simulink model "DYNctl_ver4_etud_obfusc"  (R2018b)
settings: Solver=ode45  StartTime=0.0  StopTime=tfin  FixedStep=0.001  RelTol=1e-09  EnableMultiTasking=on
values from neighbouring files (symbols this model uses):
  g = 9.81    [bancEssaiConstantes.m]
  JS = 2*mS*rS^2/5    (= 4.8672e-08)    [bancEssaiConstantes.m]
  Jxy = Jx    (= 0.001169)    [bancEssaiConstantes.m]
  L = LL    (= 0.115)    [bancEssaiConstantes.m]
  mP = 425e-03    (= 0.425)    [bancEssaiConstantes.m]
  mS = 0.0080    (= 0.008)    [bancEssaiConstantes.m]
  R = RR    (= 3.6)    [bancEssaiConstantes.m]
  rABC = 95.20e-03    (= 0.0952)    [bancEssaiConstantes.m]
  rS = 0.0039    [bancEssaiConstantes.m]
  XA = +rABC    (= 0.0952)    [bancEssaiConstantes.m]
  XB = -rABC*sind(30)    [bancEssaiConstantes.m]
  XC = -rABC*sind(30)    [bancEssaiConstantes.m]
  YA = 0.0    (= 0)    [bancEssaiConstantes.m]
  YB = +rABC*cosd(30)    [bancEssaiConstantes.m]
  YC = -rABC*cosd(30)    [bancEssaiConstantes.m]
undefined symbols (not defined in the file or in its folder): ae0, ae1, ae2, ae3, as0, as1, as2, as3, be1
settings Model: Creator=delafontaine  LastModifiedBy=Vincent
settings SolverCC: AlgebraicLoopSolver=LineSearch
settings DataIOCC: LimitDataPoints=on  SaveFormat=Array  SignalLoggingSaveFormat=ModelDataLogs
settings OptimizationCC: LifeSpan=inf
settings DebuggingCC: UnderspecifiedInitializationDetection=Classic  MergeDetectMultiDrivingBlocksExec=none  MultiTaskDSMMsg=warning  MultiTaskCondExecSysMsg=none  SFUnexpectedBacktrackingDiag=warning  SFNoUnconditionalDefaultTransitionDiag=warning  SFExecutionAtInitializationDiag=none
settings HardwareCC: ProdBitPerPointer=32  ProdBitPerSizeT=32  ProdBitPerPtrDiffT=32  ProdLargestAtomicFloat=None  ProdIntDivRoundTo=Undefined  ProdEndianess=Unspecified  ProdWordSize=32  ProdHWDeviceType=32-bit Generic
settings ModelReferenceCC: PropagateSignalLabelsOutOfModel=off
settings SFSimCC: SimUseLocalCustomCode=off
settings RTWCC: RTWUseLocalCustomCode=off
settings CodeAppCC: StateflowObjectComments=on
settings GRTTargetCC: TargetLangStandard=C89/C90 (ANSI)  GeneratePreprocessorConditionals=Disable all
settings ConfigComp: CovMetricSettings=dw  CovHtmlReporting=on  CovSaveCumulativeToWorkspaceVar=on  CovSaveSingleToWorkspaceVar=on  CovExternalEMLEnable=off  CovSFcnEnable=off

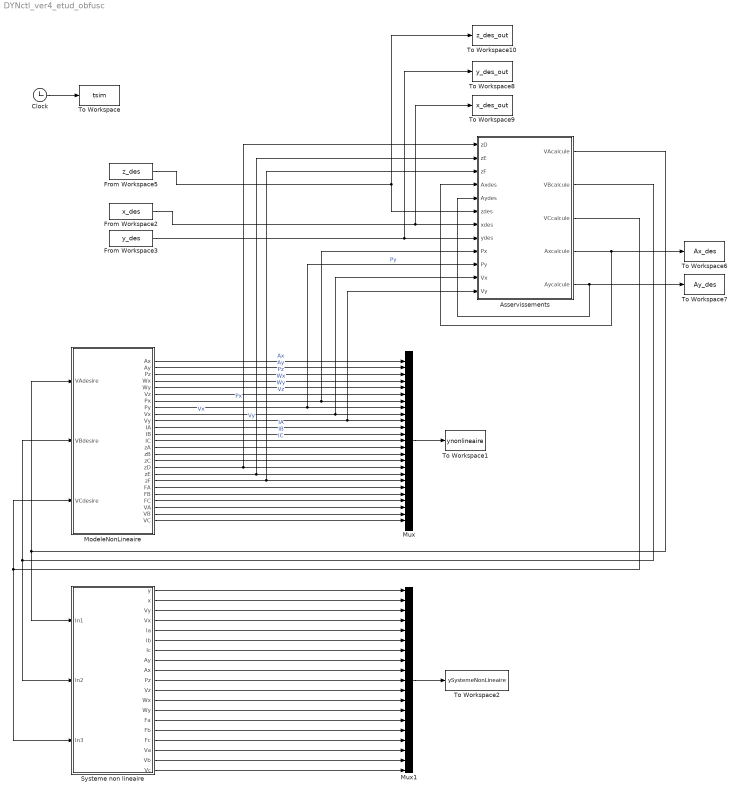
== system DYNctl_ver4_etud_obfusc ==
  Asservissements : Subsystem
      mask help: Simulink:masks:GenSFuncDesc_MD
      mask Help: eval('feval(''rtwprivate'',''rtwhelpview'',''rtw_sfcn_block'')');
  Clock : Clock
  From Workspace2 : FromWorkspace  VariableName=x_des  SampleTime=0  Interpolate=off  OutputAfterFinalValue=Holding final value
  From Workspace3 : FromWorkspace  VariableName=y_des  SampleTime=0  Interpolate=off  OutputAfterFinalValue=Holding final value
  From Workspace5 : FromWorkspace  VariableName=z_des  SampleTime=0  Interpolate=off  OutputAfterFinalValue=Holding final value
  ModeleNonLineaire : Subsystem
      mask help: Simulink:masks:GenSFuncDesc_MD
      mask Help: eval('feval(''rtwprivate'',''rtwhelpview'',''rtw_sfcn_block'')');
  Mux : Mux  Inputs=25
  Mux1 : Mux  Inputs=19
  Systeme non lineaire : Subsystem
  To Workspace : ToWorkspace  VariableName=tsim  SampleTime=-1
  To Workspace1 : ToWorkspace  VariableName=ynonlineaire  SampleTime=-1
  To Workspace10 : ToWorkspace  VariableName=z_des_out  SampleTime=-1
  To Workspace2 : ToWorkspace  VariableName=ySystemeNonLineaire  SampleTime=-1
  To Workspace6 : ToWorkspace  VariableName=Ax_des  SampleTime=-1
  To Workspace7 : ToWorkspace  VariableName=Ay_des  SampleTime=-1
  To Workspace8 : ToWorkspace  VariableName=y_des_out  SampleTime=-1
  To Workspace9 : ToWorkspace  VariableName=x_des_out  SampleTime=-1
  wires:
  Mux/1 -> To Workspace1/1
  Clock/1 -> To Workspace/1
  From Workspace5/1 -> Asservissements/6(zdes), To Workspace10/1
  ModeleNonLineaire/1(Ax) -> Mux/1  "Ax"
  ModeleNonLineaire/2(Ay) -> Mux/2  "Ay"
  ModeleNonLineaire/3(Pz) -> Mux/3  "Pz"
  ModeleNonLineaire/4(Wx) -> Mux/4  "Wx"
  ModeleNonLineaire/5(Wy) -> Mux/5  "Wy"
  ModeleNonLineaire/6(Vz) -> Mux/6  "Vz"
  ModeleNonLineaire/7(Px) -> Asservissements/9(Px), Mux/7  "Px"
  ModeleNonLineaire/8(Py) -> Asservissements/10(Py), Mux/8  "Py"
  ModeleNonLineaire/9(Vx) -> Asservissements/11(Vx), Mux/9  "Vx"
  ModeleNonLineaire/10(Vy) -> Asservissements/12(Vy), Mux/10  "Vy"
  ModeleNonLineaire/11(IA) -> Mux/11  "IA"
  ModeleNonLineaire/12(IB) -> Mux/12  "IB"
  ModeleNonLineaire/13(IC) -> Mux/13  "IC"
  From Workspace3/1 -> Asservissements/8(ydes), To Workspace8/1
  From Workspace2/1 -> Asservissements/7(xdes), To Workspace9/1
  ModeleNonLineaire/20(FA) -> Mux/20
  ModeleNonLineaire/21(FB) -> Mux/21
  ModeleNonLineaire/22(FC) -> Mux/22
  ModeleNonLineaire/23(VA) -> Mux/23
  ModeleNonLineaire/24(VB) -> Mux/24
  ModeleNonLineaire/25(VC) -> Mux/25
  ModeleNonLineaire/17(zD) -> Asservissements/1(zD), Mux/17
  ModeleNonLineaire/18(zE) -> Asservissements/2(zE), Mux/18
  ModeleNonLineaire/19(zF) -> Asservissements/3(zF), Mux/19
  ModeleNonLineaire/14(zA) -> Mux/14
  ModeleNonLineaire/15(zB) -> Mux/15
  ModeleNonLineaire/16(zC) -> Mux/16
  Asservissements/4(Axcalcule) -> Asservissements/4(Axdes), To Workspace6/1
  Asservissements/5(Aycalcule) -> Asservissements/5(Aydes), To Workspace7/1
  Asservissements/1(VAcalcule) -> Systeme non lineaire/1(In1), ModeleNonLineaire/1(VAdesire)
  Asservissements/2(VBcalcule) -> Systeme non lineaire/2(In2), ModeleNonLineaire/2(VBdesire)
  Asservissements/3(VCcalcule) -> ModeleNonLineaire/3(VCdesire), Systeme non lineaire/3(In3)
  Systeme non lineaire/4(Vx) -> Mux1/4
  Systeme non lineaire/3(Vy) -> Mux1/3
  Systeme non lineaire/2(x) -> Mux1/2
  Systeme non lineaire/1(y) -> Mux1/1
  Systeme non lineaire/5(Ia) -> Mux1/5
  Systeme non lineaire/6(Ib) -> Mux1/6
  Systeme non lineaire/7(Ic) -> Mux1/7
  Systeme non lineaire/8(Ay) -> Mux1/8
  Systeme non lineaire/9(Ax) -> Mux1/9
  Systeme non lineaire/10(Pz) -> Mux1/10
  Systeme non lineaire/11(Vz) -> Mux1/11
  Systeme non lineaire/12(Wx) -> Mux1/12
  Systeme non lineaire/13(Wy) -> Mux1/13
  Systeme non lineaire/14(Fa) -> Mux1/14
  Systeme non lineaire/15(Fb) -> Mux1/15
  Systeme non lineaire/16(Fc) -> Mux1/16
  Systeme non lineaire/17(Va) -> Mux1/17
  Systeme non lineaire/18(Vb) -> Mux1/18
  Systeme non lineaire/19(Vc) -> Mux1/19
  Mux1/1 -> To Workspace2/1

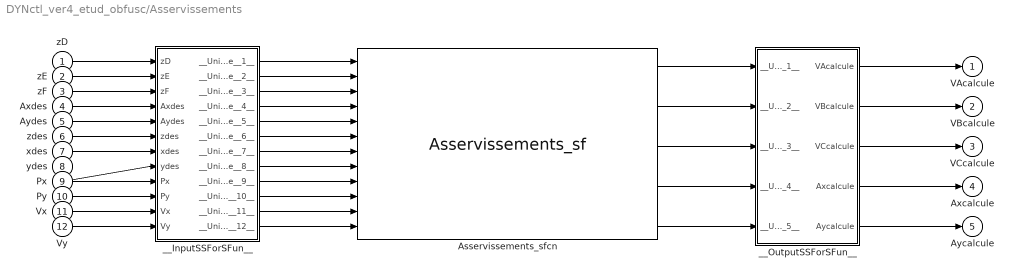
== system DYNctl_ver4_etud_obfusc/Asservissements ==
  zD : Inport
  zE : Inport  Port=2
  zF : Inport  Port=3
  Axdes : Inport  Port=4
  Aydes : Inport  Port=5
  zdes : Inport  Port=6
  xdes : Inport  Port=7
  ydes : Inport  Port=8
  Px : Inport  Port=9
  Py : Inport  Port=10
  Vx : Inport  Port=11
  Vy : Inport  Port=12
  Asservissements_sfcn : S-Function  FunctionName=Asservissements_sf  SFunctionModules=""  SFunctionDeploymentMode=off  EnableBusSupport=off  mask{rtw_sf_name=Asservissements_sf, showVar=off}
      mask prompts: rtw_sf_name "Simulink:masks:GenSFuncName_MP"; showVar "Simulink:masks:GenSFuncShowModuleList_MP"
      mask help: Simulink:masks:GenSFuncDesc_MD
      mask init:
      | displist = '';
      | if ~strcmp(get_param(gcb, 'FunctionName'), rtw_sf_name);
      |   set_param(gcb, 'FunctionName', rtw_sf_name);
      | end
      | % Check if we are generating code
      | rtw_mode = false;
      | if strcmpi(get_param(bdroot(gcb),'SimulationStatus'),'Initializing')
      | 	rtw_mode = strcmpi(get_param(bdroot(gcb),'BuildingRTWCode'),'on') && ...
      | 		~strcmpi(get_param(bdroot(gcb),'TargetStyle'),'SimulationTarget');
      | end
      | if showVar || rtw_mode
      | 	if exist('rtwsfunc') == 2 | exist('rtwsfunc') == 6
      | 		tmplist = rtwsfunc(rtw_sf_name,gcb);
      | 		tmplist = DAStudio.message('Simulink:masks:GenSFuncListOfModules_IC', tmplist);
      | 	elseif showVar
      | 		tmplist1 = DAStudio.message('Simulink:masks:GenSFuncListOfModules_IC', '');
      |         tmplist2 = DAStudio.message('Simulink:masks:GenSFuncNotLicensed_IC');
      |         tmplist = [tmplist1 tmplist2];
      |  	end
      | end
      | if showVar
      |   displist = tmplist;
      | end
      settings: CopyFcn=|
      | if ~strcmp(get_param(gcb,'Linkstatus'),'none') && ...
      | ~strcmp(get_param(gcb,'Linkstatus'),'implicit')
      |   set_param(gcb,'LinkStatus','none');
      | end
      mask Help: eval('feval(''rtwprivate'',''rtwhelpview'',''rtw_sfcn_block'')');
      mask Display:
      | port_label('input',1,'zD');
      | port_label('input',2,'zE');
      | port_label('input',3,'zF');
      | port_label('input',4,'Axdes');
      | port_label('input',5,'Aydes');
      | port_label('input',6,'zdes');
      | port_label('input',7,'xdes');
      | port_label('input',8,'ydes');
      | port_label('input',9,'Px');
      | port_label('input',10,'Py');
      | port_label('input',11,'Vx');
      | port_label('input',12,'Vy');
      | port_label('output',1,'VAcalcule');
      | port_label('output',2,'VBcalcule');
      | port_label('output',3,'VCcalcule');
      | port_label('output',4,'Axcalcule');
      | port_label('output',5,'Aycalcule');
  __InputSSForSFun__ : Subsystem
  __OutputSSForSFun__ : Subsystem
  VAcalcule : Outport
  VBcalcule : Outport  Port=2
  VCcalcule : Outport  Port=3
  Axcalcule : Outport  Port=4
  Aycalcule : Outport  Port=5
  wires:
  zD/1 -> __InputSSForSFun__/1(zD)
  zE/1 -> __InputSSForSFun__/2(zE)
  zF/1 -> __InputSSForSFun__/3(zF)
  Axdes/1 -> __InputSSForSFun__/4(Axdes)
  Aydes/1 -> __InputSSForSFun__/5(Aydes)
  zdes/1 -> __InputSSForSFun__/6(zdes)
  xdes/1 -> __InputSSForSFun__/7(xdes)
  ydes/1 -> __InputSSForSFun__/8(ydes)
  Px/1 -> __InputSSForSFun__/9(Px)
  Py/1 -> __InputSSForSFun__/10(Py)
  Vx/1 -> __InputSSForSFun__/11(Vx)
  Vy/1 -> __InputSSForSFun__/12(Vy)
  __InputSSForSFun__/1(__UniqueOutportName__1__) -> Asservissements_sfcn/1
  __InputSSForSFun__/2(__UniqueOutportName__2__) -> Asservissements_sfcn/2
  __InputSSForSFun__/3(__UniqueOutportName__3__) -> Asservissements_sfcn/3
  __InputSSForSFun__/4(__UniqueOutportName__4__) -> Asservissements_sfcn/4
  __InputSSForSFun__/5(__UniqueOutportName__5__) -> Asservissements_sfcn/5
  __InputSSForSFun__/6(__UniqueOutportName__6__) -> Asservissements_sfcn/6
  __InputSSForSFun__/7(__UniqueOutportName__7__) -> Asservissements_sfcn/7
  __InputSSForSFun__/8(__UniqueOutportName__8__) -> Asservissements_sfcn/8
  __InputSSForSFun__/9(__UniqueOutportName__9__) -> Asservissements_sfcn/9
  __InputSSForSFun__/10(__UniqueOutportName__10__) -> Asservissements_sfcn/10
  __InputSSForSFun__/11(__UniqueOutportName__11__) -> Asservissements_sfcn/11
  __InputSSForSFun__/12(__UniqueOutportName__12__) -> Asservissements_sfcn/12
  Asservissements_sfcn/1 -> __OutputSSForSFun__/1(__UniqueInportName__1__)
  Asservissements_sfcn/2 -> __OutputSSForSFun__/2(__UniqueInportName__2__)
  Asservissements_sfcn/3 -> __OutputSSForSFun__/3(__UniqueInportName__3__)
  Asservissements_sfcn/4 -> __OutputSSForSFun__/4(__UniqueInportName__4__)
  Asservissements_sfcn/5 -> __OutputSSForSFun__/5(__UniqueInportName__5__)
  __OutputSSForSFun__/1(VAcalcule) -> VAcalcule/1
  __OutputSSForSFun__/2(VBcalcule) -> VBcalcule/1
  __OutputSSForSFun__/3(VCcalcule) -> VCcalcule/1
  __OutputSSForSFun__/4(Axcalcule) -> Axcalcule/1
  __OutputSSForSFun__/5(Aycalcule) -> Aycalcule/1

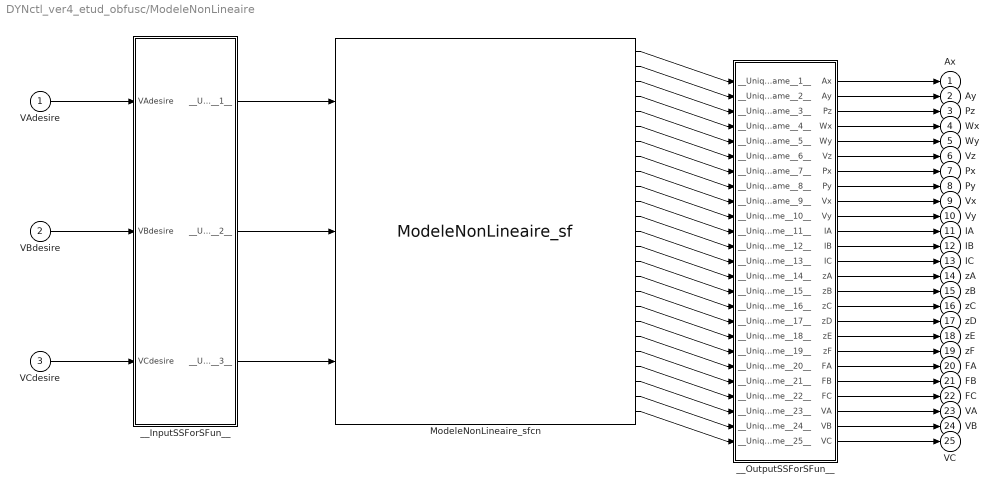
== system DYNctl_ver4_etud_obfusc/ModeleNonLineaire ==
  VAdesire : Inport
  VBdesire : Inport  Port=2
  VCdesire : Inport  Port=3
  ModeleNonLineaire_sfcn : S-Function  FunctionName=ModeleNonLineaire_sf  SFunctionModules=""  SFunctionDeploymentMode=off  EnableBusSupport=off  mask{rtw_sf_name=ModeleNonLineaire_sf, showVar=off}
      mask prompts: rtw_sf_name "Simulink:masks:GenSFuncName_MP"; showVar "Simulink:masks:GenSFuncShowModuleList_MP"
      mask help: Simulink:masks:GenSFuncDesc_MD
      mask init: same as DYNctl_ver4_etud_obfusc/Asservissements/Asservissements_sfcn
      settings: CopyFcn=|
      | if ~strcmp(get_param(gcb,'Linkstatus'),'none') && ...
      | ~strcmp(get_param(gcb,'Linkstatus'),'implicit')
      |   set_param(gcb,'LinkStatus','none');
      | end
      mask Help: eval('feval(''rtwprivate'',''rtwhelpview'',''rtw_sfcn_block'')');
      mask Display:
      | port_label('input',1,'VAdesire');
      | port_label('input',2,'VBdesire');
      | port_label('input',3,'VCdesire');
      | port_label('output',1,'Ax');
      | port_label('output',2,'Ay');
      | port_label('output',3,'Pz');
      | port_label('output',4,'Wx');
      | port_label('output',5,'Wy');
      | port_label('output',6,'Vz');
      | port_label('output',7,'Px');
      | port_label('output',8,'Py');
      | port_label('output',9,'Vx');
      | port_label('output',10,'Vy');
      | port_label('output',11,'IA');
      | port_label('output',12,'IB');
      | port_label('output',13,'IC');
      | port_label('output',14,'zA');
      | port_label('output',15,'zB');
      | port_label('output',16,'zC');
      | port_label('output',17,'zD');
      | port_label('output',18,'zE');
      | port_label('output',19,'zF');
      | port_label('output',20,'FA');
      | port_label('output',21,'FB');
      | port_label('output',22,'FC');
      | port_label('output',23,'VA');
      | port_label('output',24,'VB');
      | port_label('output',25,'VC');
  __InputSSForSFun__ : Subsystem
  __OutputSSForSFun__ : Subsystem
  Ax : Outport
  Ay : Outport  Port=2
  Pz : Outport  Port=3
  Wx : Outport  Port=4
  Wy : Outport  Port=5
  Vz : Outport  Port=6
  Px : Outport  Port=7
  Py : Outport  Port=8
  Vx : Outport  Port=9
  Vy : Outport  Port=10
  IA : Outport  Port=11
  IB : Outport  Port=12
  IC : Outport  Port=13
  zA : Outport  Port=14
  zB : Outport  Port=15
  zC : Outport  Port=16
  zD : Outport  Port=17
  zE : Outport  Port=18
  zF : Outport  Port=19
  FA : Outport  Port=20
  FB : Outport  Port=21
  FC : Outport  Port=22
  VA : Outport  Port=23
  VB : Outport  Port=24
  VC : Outport  Port=25
  wires:
  VAdesire/1 -> __InputSSForSFun__/1(VAdesire)
  VBdesire/1 -> __InputSSForSFun__/2(VBdesire)
  VCdesire/1 -> __InputSSForSFun__/3(VCdesire)
  __InputSSForSFun__/1(__UniqueOutportName__1__) -> ModeleNonLineaire_sfcn/1
  __InputSSForSFun__/2(__UniqueOutportName__2__) -> ModeleNonLineaire_sfcn/2
  __InputSSForSFun__/3(__UniqueOutportName__3__) -> ModeleNonLineaire_sfcn/3
  ModeleNonLineaire_sfcn/1 -> __OutputSSForSFun__/1(__UniqueInportName__1__)
  ModeleNonLineaire_sfcn/2 -> __OutputSSForSFun__/2(__UniqueInportName__2__)
  ModeleNonLineaire_sfcn/3 -> __OutputSSForSFun__/3(__UniqueInportName__3__)
  ModeleNonLineaire_sfcn/4 -> __OutputSSForSFun__/4(__UniqueInportName__4__)
  ModeleNonLineaire_sfcn/5 -> __OutputSSForSFun__/5(__UniqueInportName__5__)
  ModeleNonLineaire_sfcn/6 -> __OutputSSForSFun__/6(__UniqueInportName__6__)
  ModeleNonLineaire_sfcn/7 -> __OutputSSForSFun__/7(__UniqueInportName__7__)
  ModeleNonLineaire_sfcn/8 -> __OutputSSForSFun__/8(__UniqueInportName__8__)
  ModeleNonLineaire_sfcn/9 -> __OutputSSForSFun__/9(__UniqueInportName__9__)
  ModeleNonLineaire_sfcn/10 -> __OutputSSForSFun__/10(__UniqueInportName__10__)
  ModeleNonLineaire_sfcn/11 -> __OutputSSForSFun__/11(__UniqueInportName__11__)
  ModeleNonLineaire_sfcn/12 -> __OutputSSForSFun__/12(__UniqueInportName__12__)
  ModeleNonLineaire_sfcn/13 -> __OutputSSForSFun__/13(__UniqueInportName__13__)
  ModeleNonLineaire_sfcn/14 -> __OutputSSForSFun__/14(__UniqueInportName__14__)
  ModeleNonLineaire_sfcn/15 -> __OutputSSForSFun__/15(__UniqueInportName__15__)
  ModeleNonLineaire_sfcn/16 -> __OutputSSForSFun__/16(__UniqueInportName__16__)
  ModeleNonLineaire_sfcn/17 -> __OutputSSForSFun__/17(__UniqueInportName__17__)
  ModeleNonLineaire_sfcn/18 -> __OutputSSForSFun__/18(__UniqueInportName__18__)
  ModeleNonLineaire_sfcn/19 -> __OutputSSForSFun__/19(__UniqueInportName__19__)
  ModeleNonLineaire_sfcn/20 -> __OutputSSForSFun__/20(__UniqueInportName__20__)
  ModeleNonLineaire_sfcn/21 -> __OutputSSForSFun__/21(__UniqueInportName__21__)
  ModeleNonLineaire_sfcn/22 -> __OutputSSForSFun__/22(__UniqueInportName__22__)
  ModeleNonLineaire_sfcn/23 -> __OutputSSForSFun__/23(__UniqueInportName__23__)
  ModeleNonLineaire_sfcn/24 -> __OutputSSForSFun__/24(__UniqueInportName__24__)
  ModeleNonLineaire_sfcn/25 -> __OutputSSForSFun__/25(__UniqueInportName__25__)
  __OutputSSForSFun__/1(Ax) -> Ax/1
  __OutputSSForSFun__/2(Ay) -> Ay/1
  __OutputSSForSFun__/3(Pz) -> Pz/1
  __OutputSSForSFun__/4(Wx) -> Wx/1
  __OutputSSForSFun__/5(Wy) -> Wy/1
  __OutputSSForSFun__/6(Vz) -> Vz/1
  __OutputSSForSFun__/7(Px) -> Px/1
  __OutputSSForSFun__/8(Py) -> Py/1
  __OutputSSForSFun__/9(Vx) -> Vx/1
  __OutputSSForSFun__/10(Vy) -> Vy/1
  __OutputSSForSFun__/11(IA) -> IA/1
  __OutputSSForSFun__/12(IB) -> IB/1
  __OutputSSForSFun__/13(IC) -> IC/1
  __OutputSSForSFun__/14(zA) -> zA/1
  __OutputSSForSFun__/15(zB) -> zB/1
  __OutputSSForSFun__/16(zC) -> zC/1
  __OutputSSForSFun__/17(zD) -> zD/1
  __OutputSSForSFun__/18(zE) -> zE/1
  __OutputSSForSFun__/19(zF) -> zF/1
  __OutputSSForSFun__/20(FA) -> FA/1
  __OutputSSForSFun__/21(FB) -> FB/1
  __OutputSSForSFun__/22(FC) -> FC/1
  __OutputSSForSFun__/23(VA) -> VA/1
  __OutputSSForSFun__/24(VB) -> VB/1
  __OutputSSForSFun__/25(VC) -> VC/1

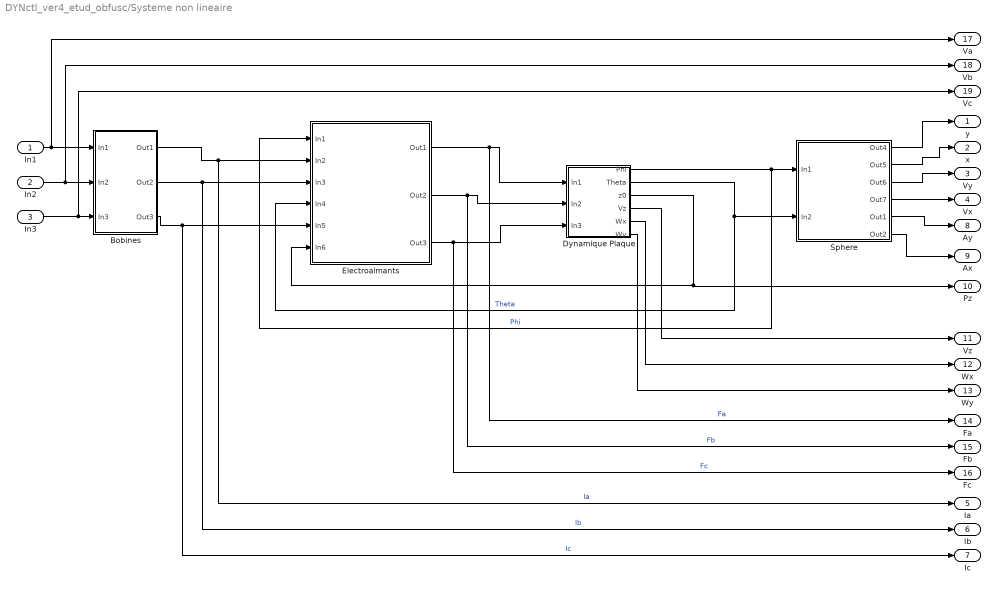
== system DYNctl_ver4_etud_obfusc/Systeme non lineaire ==
  In1 : Inport
  In2 : Inport  Port=2
  In3 : Inport  Port=3
  Bobines : Subsystem
  Dynamique Plaque : Subsystem
  Electroaimants : Subsystem
  Sphere : Subsystem
  y : Outport
  x : Outport  Port=2
  Vy : Outport  Port=3
  Vx : Outport  Port=4
  Ia : Outport  Port=5
  Ib : Outport  Port=6
  Ic : Outport  Port=7
  Ay : Outport  Port=8
  Ax : Outport  Port=9
  Pz : Outport  Port=10
  Vz : Outport  Port=11
  Wx : Outport  Port=12
  Wy : Outport  Port=13
  Fa : Outport  Port=14
  Fb : Outport  Port=15
  Fc : Outport  Port=16
  Va : Outport  Port=17
  Vb : Outport  Port=18
  Vc : Outport  Port=19
  wires:
  Electroaimants/2(Out2) -> Fb/1, Dynamique Plaque/2(In2)  "Fb"
  Bobines/2(Out2) -> Ib/1, Electroaimants/3(In3)  "Ib"
  Bobines/1(Out1) -> Ia/1, Electroaimants/2(In2)  "Ia"
  Dynamique Plaque/2(Theta) -> Electroaimants/4(In4), Sphere/2(In2)  "Theta"
  In2/1 -> Vb/1, Bobines/2(In2)
  Electroaimants/1(Out1) -> Fa/1, Dynamique Plaque/1(In1)  "Fa"
  In1/1 -> Bobines/1(In1), Va/1
  Electroaimants/3(Out3) -> Fc/1, Dynamique Plaque/3(In3)  "Fc"
  Dynamique Plaque/1(Phi) -> Electroaimants/1(In1), Sphere/1(In1)  "Phi"
  Bobines/3(Out3) -> Ic/1, Electroaimants/5(In5)  "Ic"
  Dynamique Plaque/3(z0) -> Electroaimants/6(In6), Pz/1
  In3/1 -> Vc/1, Bobines/3(In3)
  Sphere/1(Out4) -> y/1
  Sphere/2(Out5) -> x/1
  Sphere/3(Out6) -> Vy/1
  Sphere/4(Out7) -> Vx/1
  Sphere/5(Out1) -> Ay/1
  Sphere/6(Out2) -> Ax/1
  Dynamique Plaque/4(Vz) -> Vz/1
  Dynamique Plaque/5(Wx) -> Wx/1
  Dynamique Plaque/6(Wy) -> Wy/1

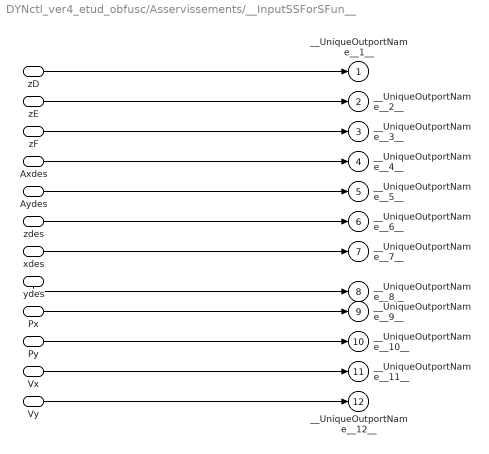
== system DYNctl_ver4_etud_obfusc/Asservissements/__InputSSForSFun__ ==
  zD : Inport
  zE : Inport  Port=2
  zF : Inport  Port=3
  Axdes : Inport  Port=4
  Aydes : Inport  Port=5
  zdes : Inport  Port=6
  xdes : Inport  Port=7
  ydes : Inport  Port=8
  Px : Inport  Port=9
  Py : Inport  Port=10
  Vx : Inport  Port=11
  Vy : Inport  Port=12
  __UniqueOutportName__1__ : Outport
  __UniqueOutportName__2__ : Outport  Port=2
  __UniqueOutportName__3__ : Outport  Port=3
  __UniqueOutportName__4__ : Outport  Port=4
  __UniqueOutportName__5__ : Outport  Port=5
  __UniqueOutportName__6__ : Outport  Port=6
  __UniqueOutportName__7__ : Outport  Port=7
  __UniqueOutportName__8__ : Outport  Port=8
  __UniqueOutportName__9__ : Outport  Port=9
  __UniqueOutportName__10__ : Outport  Port=10
  __UniqueOutportName__11__ : Outport  Port=11
  __UniqueOutportName__12__ : Outport  Port=12
  wires:
  zD/1 -> __UniqueOutportName__1__/1
  zE/1 -> __UniqueOutportName__2__/1
  zF/1 -> __UniqueOutportName__3__/1
  Axdes/1 -> __UniqueOutportName__4__/1
  Aydes/1 -> __UniqueOutportName__5__/1
  zdes/1 -> __UniqueOutportName__6__/1
  xdes/1 -> __UniqueOutportName__7__/1
  ydes/1 -> __UniqueOutportName__8__/1
  Px/1 -> __UniqueOutportName__9__/1
  Py/1 -> __UniqueOutportName__10__/1
  Vx/1 -> __UniqueOutportName__11__/1
  Vy/1 -> __UniqueOutportName__12__/1

== system DYNctl_ver4_etud_obfusc/Asservissements/__OutputSSForSFun__ ==
  __UniqueInportName__1__ : Inport
  __UniqueInportName__2__ : Inport  Port=2
  __UniqueInportName__3__ : Inport  Port=3
  __UniqueInportName__4__ : Inport  Port=4
  __UniqueInportName__5__ : Inport  Port=5
  VAcalcule : Outport
  VBcalcule : Outport  Port=2
  VCcalcule : Outport  Port=3
  Axcalcule : Outport  Port=4
  Aycalcule : Outport  Port=5
  wires:
  __UniqueInportName__1__/1 -> VAcalcule/1
  __UniqueInportName__2__/1 -> VBcalcule/1
  __UniqueInportName__3__/1 -> VCcalcule/1
  __UniqueInportName__4__/1 -> Axcalcule/1  "Ax_des"
  __UniqueInportName__5__/1 -> Aycalcule/1  "Ay_des"

== system DYNctl_ver4_etud_obfusc/ModeleNonLineaire/__InputSSForSFun__ ==
  VAdesire : Inport
  VBdesire : Inport  Port=2
  VCdesire : Inport  Port=3
  __UniqueOutportName__1__ : Outport
  __UniqueOutportName__2__ : Outport  Port=2
  __UniqueOutportName__3__ : Outport  Port=3
  wires:
  VAdesire/1 -> __UniqueOutportName__1__/1
  VBdesire/1 -> __UniqueOutportName__2__/1
  VCdesire/1 -> __UniqueOutportName__3__/1

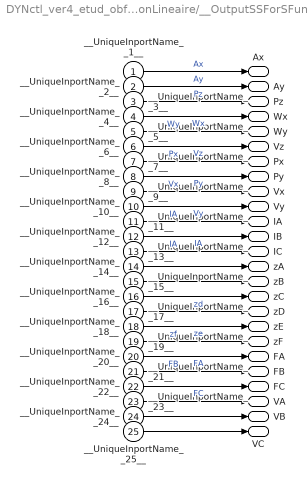
== system DYNctl_ver4_etud_obfusc/ModeleNonLineaire/__OutputSSForSFun__ ==
  __UniqueInportName__1__ : Inport
  __UniqueInportName__2__ : Inport  Port=2
  __UniqueInportName__3__ : Inport  Port=3
  __UniqueInportName__4__ : Inport  Port=4
  __UniqueInportName__5__ : Inport  Port=5
  __UniqueInportName__6__ : Inport  Port=6
  __UniqueInportName__7__ : Inport  Port=7
  __UniqueInportName__8__ : Inport  Port=8
  __UniqueInportName__9__ : Inport  Port=9
  __UniqueInportName__10__ : Inport  Port=10
  __UniqueInportName__11__ : Inport  Port=11
  __UniqueInportName__12__ : Inport  Port=12
  __UniqueInportName__13__ : Inport  Port=13
  __UniqueInportName__14__ : Inport  Port=14
  __UniqueInportName__15__ : Inport  Port=15
  __UniqueInportName__16__ : Inport  Port=16
  __UniqueInportName__17__ : Inport  Port=17
  __UniqueInportName__18__ : Inport  Port=18
  __UniqueInportName__19__ : Inport  Port=19
  __UniqueInportName__20__ : Inport  Port=20
  __UniqueInportName__21__ : Inport  Port=21
  __UniqueInportName__22__ : Inport  Port=22
  __UniqueInportName__23__ : Inport  Port=23
  __UniqueInportName__24__ : Inport  Port=24
  __UniqueInportName__25__ : Inport  Port=25
  Ax : Outport
  Ay : Outport  Port=2
  Pz : Outport  Port=3
  Wx : Outport  Port=4
  Wy : Outport  Port=5
  Vz : Outport  Port=6
  Px : Outport  Port=7
  Py : Outport  Port=8
  Vx : Outport  Port=9
  Vy : Outport  Port=10
  IA : Outport  Port=11
  IB : Outport  Port=12
  IC : Outport  Port=13
  zA : Outport  Port=14
  zB : Outport  Port=15
  zC : Outport  Port=16
  zD : Outport  Port=17
  zE : Outport  Port=18
  zF : Outport  Port=19
  FA : Outport  Port=20
  FB : Outport  Port=21
  FC : Outport  Port=22
  VA : Outport  Port=23
  VB : Outport  Port=24
  VC : Outport  Port=25
  wires:
  __UniqueInportName__1__/1 -> Ax/1  "Ax"
  __UniqueInportName__2__/1 -> Ay/1  "Ay"
  __UniqueInportName__3__/1 -> Pz/1  "Pz"
  __UniqueInportName__4__/1 -> Wx/1  "Wx"
  __UniqueInportName__5__/1 -> Wy/1  "Wy"
  __UniqueInportName__6__/1 -> Vz/1  "Vz"
  __UniqueInportName__7__/1 -> Px/1  "Px"
  __UniqueInportName__8__/1 -> Py/1  "Py"
  __UniqueInportName__9__/1 -> Vx/1  "Vx"
  __UniqueInportName__10__/1 -> Vy/1  "Vy"
  __UniqueInportName__11__/1 -> IA/1  "IA"
  __UniqueInportName__12__/1 -> IB/1  "IA"
  __UniqueInportName__13__/1 -> IC/1  "IA"
  __UniqueInportName__14__/1 -> zA/1
  __UniqueInportName__15__/1 -> zB/1
  __UniqueInportName__16__/1 -> zC/1
  __UniqueInportName__17__/1 -> zD/1  "zd"
  __UniqueInportName__18__/1 -> zE/1  "ze"
  __UniqueInportName__19__/1 -> zF/1  "zf"
  __UniqueInportName__20__/1 -> FA/1  "FA"
  __UniqueInportName__21__/1 -> FB/1  "FB"
  __UniqueInportName__22__/1 -> FC/1  "FC"
  __UniqueInportName__23__/1 -> VA/1
  __UniqueInportName__24__/1 -> VB/1
  __UniqueInportName__25__/1 -> VC/1

== system DYNctl_ver4_etud_obfusc/Systeme non lineaire/Bobines ==
  In1 : Inport
  In2 : Inport  Port=2
  In3 : Inport  Port=3
  Subsystem : Subsystem
  Subsystem1 : Subsystem
  Subsystem2 : Subsystem
  Out1 : Outport
  Out2 : Outport  Port=2
  Out3 : Outport  Port=3
  wires:
  In1/1 -> Subsystem/1(In1)  "Va"
  In2/1 -> Subsystem1/1(In1)  "Vb"
  Subsystem2/1(Out1) -> Out3/1  "Ic"
  Subsystem/1(Out1) -> Out1/1  "Ia"
  In3/1 -> Subsystem2/1(In1)  "Vc"
  Subsystem1/1(Out1) -> Out2/1  "Ib"

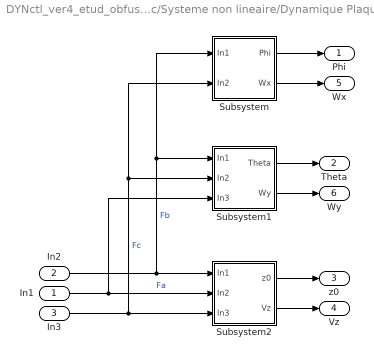
== system DYNctl_ver4_etud_obfusc/Systeme non lineaire/Dynamique Plaque ==
  In1 : Inport
  In2 : Inport  Port=2
  In3 : Inport  Port=3
  Subsystem : Subsystem
  Subsystem1 : Subsystem
  Subsystem2 : Subsystem
  Phi : Outport
  Theta : Outport  Port=2
  z0 : Outport  Port=3
  Vz : Outport  Port=4
  Wx : Outport  Port=5
  Wy : Outport  Port=6
  wires:
  In1/1 -> Subsystem1/3(In3), Subsystem2/2(In2)  "Fa"
  In3/1 -> Subsystem/2(In2), Subsystem1/2(In2), Subsystem2/3(In3)  "Fc"
  Subsystem1/1(Theta) -> Theta/1
  In2/1 -> Subsystem1/1(In1), Subsystem/1(In1), Subsystem2/1(In1)  "Fb"
  Subsystem/1(Phi) -> Phi/1
  Subsystem2/1(z0) -> z0/1
  Subsystem2/2(Vz) -> Vz/1
  Subsystem/2(Wx) -> Wx/1
  Subsystem1/2(Wy) -> Wy/1

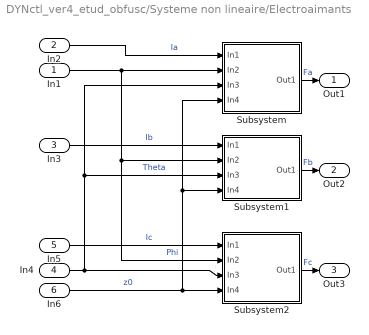
== system DYNctl_ver4_etud_obfusc/Systeme non lineaire/Electroaimants ==
  In1 : Inport
  In2 : Inport  Port=2
  In3 : Inport  Port=3
  In4 : Inport  Port=4
  In5 : Inport  Port=5
  In6 : Inport  Port=6
  Subsystem : Subsystem
  Subsystem1 : Subsystem
  Subsystem2 : Subsystem
  Out1 : Outport
  Out2 : Outport  Port=2
  Out3 : Outport  Port=3
  wires:
  In6/1 -> Subsystem2/4(In4), Subsystem1/4(In4), Subsystem/4(In4)  "z0"
  In4/1 -> Subsystem2/3(In3), Subsystem/3(In3), Subsystem1/3(In3)  "Theta"
  In5/1 -> Subsystem2/1(In1)  "Ic"
  In1/1 -> Subsystem/2(In2), Subsystem2/2(In2), Subsystem1/2(In2)  "Phi"
  Subsystem2/1(Out1) -> Out3/1  "Fc"
  In2/1 -> Subsystem/1(In1)  "Ia"
  In3/1 -> Subsystem1/1(In1)  "Ib"
  Subsystem1/1(Out1) -> Out2/1  "Fb"
  Subsystem/1(Out1) -> Out1/1  "Fa"

== system DYNctl_ver4_etud_obfusc/Systeme non lineaire/Sphere ==
  In1 : Inport
  In2 : Inport  Port=2
  Gain : Gain  Gain=-1
  Subsystem3 : Subsystem
  Subsystem4 : Subsystem
  Out4 : Outport
  Out5 : Outport  Port=2
  Out6 : Outport  Port=3
  Out7 : Outport  Port=4
  Out1 : Outport  Port=5
  Out2 : Outport  Port=6
  wires:
  Subsystem3/2(Out1) -> Out6/1  "Vy"
  Subsystem4/1(Out4) -> Out5/1  "x"
  Subsystem3/1(Out4) -> Out4/1  "y"
  In2/1 -> Gain/1
  Subsystem4/2(Out1) -> Out7/1  "Vx"
  Gain/1 -> Subsystem4/1(In4)
  In1/1 -> Subsystem3/1(In4)  "Phi"
  Subsystem3/3(Out2) -> Out1/1  "Ay"
  Subsystem4/3(Out2) -> Out2/1

== system DYNctl_ver4_etud_obfusc/Systeme non lineaire/Bobines/Subsystem ==
  note: Ia
  note: Va
  In1 : Inport
  Gain : Gain  Gain=L
  Gain1 : Gain  Gain=R/L
  Integrator : Integrator
  Sum : Sum  Inputs=|+-
  Out1 : Outport
  wires:
  Integrator/1 -> Out1/1, Gain1/1
  Gain/1 -> Sum/1
  Gain1/1 -> Sum/2
  Sum/1 -> Integrator/1
  In1/1 -> Gain/1

== system DYNctl_ver4_etud_obfusc/Systeme non lineaire/Bobines/Subsystem1 ==
  In1 : Inport
  Gain : Gain  Gain=L
  Gain1 : Gain  Gain=R/L
  Integrator : Integrator
  Sum : Sum  Inputs=|+-
  Out1 : Outport
  wires:
  Integrator/1 -> Out1/1, Gain1/1
  Gain/1 -> Sum/1
  Gain1/1 -> Sum/2
  Sum/1 -> Integrator/1
  In1/1 -> Gain/1

== system DYNctl_ver4_etud_obfusc/Systeme non lineaire/Bobines/Subsystem2 ==
  In1 : Inport
  Gain : Gain  Gain=L
  Gain1 : Gain  Gain=R/L
  Integrator : Integrator
  Sum : Sum  Inputs=|+-
  Out1 : Outport
  wires:
  Integrator/1 -> Out1/1, Gain1/1
  Gain/1 -> Sum/1
  Gain1/1 -> Sum/2
  Sum/1 -> Integrator/1
  In1/1 -> Gain/1

== system DYNctl_ver4_etud_obfusc/Systeme non lineaire/Dynamique Plaque/Subsystem ==
  In1 : Inport
  In2 : Inport  Port=2
  Gain10 : Gain  Gain=rABC*cosd(30)
  Gain11 : Gain  Gain=rABC*cosd(30)
  Gain12 : Gain  Gain=1/Jxy
  Integrator : Integrator
  Integrator1 : Integrator
  Sum9 : Sum  Inputs=|+-
  Phi : Outport
  Wx : Outport  Port=2
  wires:
  Integrator1/1 -> Phi/1
  In2/1 -> Gain11/1
  Integrator/1 -> Wx/1, Integrator1/1
  Gain10/1 -> Sum9/1
  Sum9/1 -> Gain12/1
  Gain12/1 -> Integrator/1
  Gain11/1 -> Sum9/2
  In1/1 -> Gain10/1

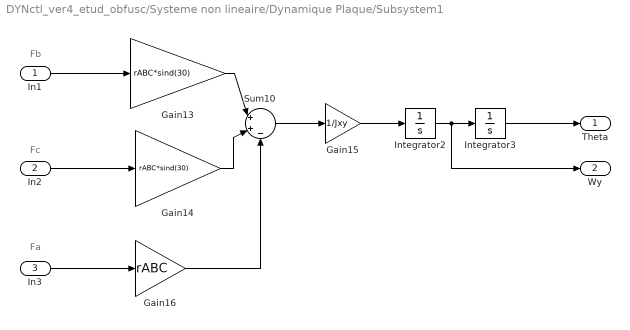
== system DYNctl_ver4_etud_obfusc/Systeme non lineaire/Dynamique Plaque/Subsystem1 ==
  note: Fa
  note: Fc
  note: Fb
  In1 : Inport
  In2 : Inport  Port=2
  In3 : Inport  Port=3
  Gain13 : Gain  Gain=rABC*sind(30)
  Gain14 : Gain  Gain=rABC*sind(30)
  Gain15 : Gain  Gain=1/Jxy
  Gain16 : Gain  Gain=rABC
  Integrator2 : Integrator
  Integrator3 : Integrator
  Sum10 : Sum  Inputs=|++-
  Theta : Outport
  Wy : Outport  Port=2
  wires:
  In3/1 -> Gain16/1
  Gain14/1 -> Sum10/2
  Gain15/1 -> Integrator2/1
  Sum10/1 -> Gain15/1
  Integrator2/1 -> Wy/1, Integrator3/1
  In1/1 -> Gain13/1
  Gain13/1 -> Sum10/1
  Integrator3/1 -> Theta/1
  Gain16/1 -> Sum10/3
  In2/1 -> Gain14/1

== system DYNctl_ver4_etud_obfusc/Systeme non lineaire/Dynamique Plaque/Subsystem2 ==
  note: Fc
  note: Fa
  note: Fb
  In1 : Inport
  In2 : Inport  Port=2
  In3 : Inport  Port=3
  Constant3 : Constant  Value=g
  Gain17 : Gain  Gain=1/mP
  Integrator4 : Integrator
  Integrator5 : Integrator
  Sum11 : Sum  Inputs=|+++
  Sum12 : Sum  Inputs=|++
  z0 : Outport
  Vz : Outport  Port=2
  wires:
  Integrator5/1 -> z0/1  "z0"
  Gain17/1 -> Sum12/1
  In3/1 -> Sum11/3
  Sum11/1 -> Gain17/1
  Constant3/1 -> Sum12/2
  In1/1 -> Sum11/2
  Integrator4/1 -> Vz/1, Integrator5/1
  Sum12/1 -> Integrator4/1
  In2/1 -> Sum11/1

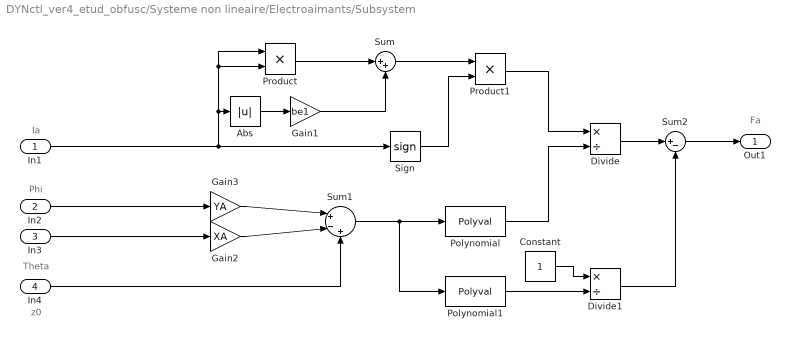
== system DYNctl_ver4_etud_obfusc/Systeme non lineaire/Electroaimants/Subsystem ==
  note: Fa
  note: z0
  note: Theta
  note: Phi
  note: Ia
  In1 : Inport
  In2 : Inport  Port=2
  In3 : Inport  Port=3
  In4 : Inport  Port=4
  Abs : Abs
  Constant : Constant
  Divide : Product  Inputs=*/
  Divide1 : Product  Inputs=*/
  Gain1 : Gain  Gain=be1
  Gain2 : Gain  Gain=XA
  Gain3 : Gain  Gain=YA
  Polynomial : Polyval  Coefs=[ae3 ae2 ae1 ae0]
  Polynomial1 : Polyval  Coefs=[as3 as2 as1 as0]
  Product : Product
  Product1 : Product
  Sign : Signum
  Sum : Sum  Inputs=|++
  Sum1 : Sum  Inputs=|+-+
  Sum2 : Sum  Inputs=|+-
  Out1 : Outport
  wires:
  Sum/1 -> Product1/1
  Product1/1 -> Divide/1
  Gain2/1 -> Sum1/2
  Sum2/1 -> Out1/1
  Constant/1 -> Divide1/1
  Product/1 -> Sum/1
  Polynomial/1 -> Divide/2
  In1/1 -> Product/1, Product/2, Abs/1, Sign/1
  Abs/1 -> Gain1/1
  Gain1/1 -> Sum/2
  Polynomial1/1 -> Divide1/2
  Sum1/1 -> Polynomial1/1, Polynomial/1
  Sign/1 -> Product1/2
  In4/1 -> Sum1/3
  Divide/1 -> Sum2/1
  Gain3/1 -> Sum1/1
  Divide1/1 -> Sum2/2
  In2/1 -> Gain3/1
  In3/1 -> Gain2/1

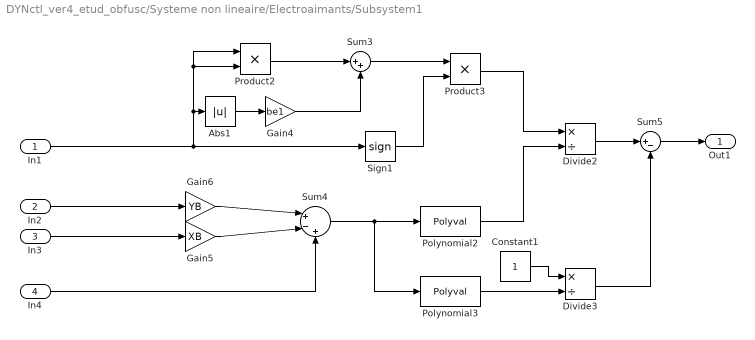
== system DYNctl_ver4_etud_obfusc/Systeme non lineaire/Electroaimants/Subsystem1 ==
  In1 : Inport
  In2 : Inport  Port=2
  In3 : Inport  Port=3
  In4 : Inport  Port=4
  Abs1 : Abs
  Constant1 : Constant
  Divide2 : Product  Inputs=*/
  Divide3 : Product  Inputs=*/
  Gain4 : Gain  Gain=be1
  Gain5 : Gain  Gain=XB
  Gain6 : Gain  Gain=YB
  Polynomial2 : Polyval  Coefs=[ae3 ae2 ae1 ae0]
  Polynomial3 : Polyval  Coefs=[as3 as2 as1 as0]
  Product2 : Product
  Product3 : Product
  Sign1 : Signum
  Sum3 : Sum  Inputs=|++
  Sum4 : Sum  Inputs=|+-+
  Sum5 : Sum  Inputs=|+-
  Out1 : Outport
  wires:
  In2/1 -> Gain6/1
  Gain6/1 -> Sum4/1
  In4/1 -> Sum4/3
  Gain5/1 -> Sum4/2
  Sum4/1 -> Polynomial3/1, Polynomial2/1
  In1/1 -> Product2/1, Product2/2, Abs1/1, Sign1/1
  Constant1/1 -> Divide3/1
  Sign1/1 -> Product3/2
  Divide2/1 -> Sum5/1
  In3/1 -> Gain5/1
  Divide3/1 -> Sum5/2
  Polynomial3/1 -> Divide3/2
  Product3/1 -> Divide2/1
  Gain4/1 -> Sum3/2
  Abs1/1 -> Gain4/1
  Product2/1 -> Sum3/1
  Sum3/1 -> Product3/1
  Polynomial2/1 -> Divide2/2
  Sum5/1 -> Out1/1

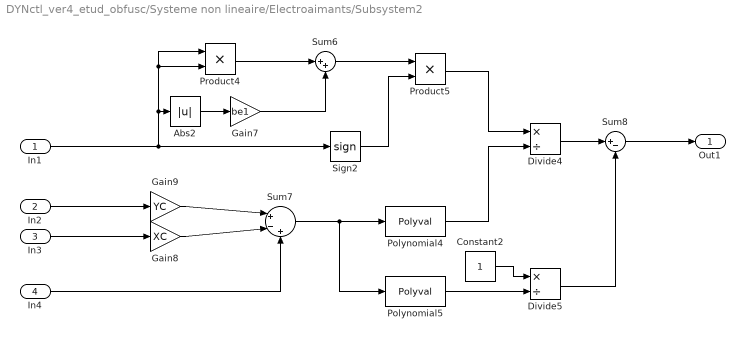
== system DYNctl_ver4_etud_obfusc/Systeme non lineaire/Electroaimants/Subsystem2 ==
  In1 : Inport
  In2 : Inport  Port=2
  In3 : Inport  Port=3
  In4 : Inport  Port=4
  Abs2 : Abs
  Constant2 : Constant
  Divide4 : Product  Inputs=*/
  Divide5 : Product  Inputs=*/
  Gain7 : Gain  Gain=be1
  Gain8 : Gain  Gain=XC
  Gain9 : Gain  Gain=YC
  Polynomial4 : Polyval  Coefs=[ae3 ae2 ae1 ae0]
  Polynomial5 : Polyval  Coefs=[as3 as2 as1 as0]
  Product4 : Product
  Product5 : Product
  Sign2 : Signum
  Sum6 : Sum  Inputs=|++
  Sum7 : Sum  Inputs=|+-+
  Sum8 : Sum  Inputs=|+-
  Out1 : Outport
  wires:
  Gain9/1 -> Sum7/1
  Gain8/1 -> Sum7/2
  Divide5/1 -> Sum8/2
  Divide4/1 -> Sum8/1
  Constant2/1 -> Divide5/1
  In1/1 -> Product4/1, Product4/2, Abs2/1, Sign2/1
  Sum7/1 -> Polynomial5/1, Polynomial4/1
  Sign2/1 -> Product5/2
  In2/1 -> Gain9/1
  Product4/1 -> Sum6/1
  Product5/1 -> Divide4/1
  In4/1 -> Sum7/3
  Polynomial5/1 -> Divide5/2
  Gain7/1 -> Sum6/2
  Polynomial4/1 -> Divide4/2
  Sum6/1 -> Product5/1
  Abs2/1 -> Gain7/1
  Sum8/1 -> Out1/1
  In3/1 -> Gain8/1

== system DYNctl_ver4_etud_obfusc/Systeme non lineaire/Sphere/Subsystem3 ==
  note: Ay
  note: y
  note: Vy
  note: Phi
  In4 : Inport  Tag=Theta
  Gain : Gain  Gain=mS*g/(mS+JS/rS^2)
  Integrator : Integrator
  Integrator1 : Integrator
  Out4 : Outport
  Out1 : Outport  Port=2
  Out2 : Outport  Port=3
  wires:
  Gain/1 -> Out2/1, Integrator/1
  In4/1 -> Gain/1
  Integrator1/1 -> Out4/1
  Integrator/1 -> Out1/1, Integrator1/1

== system DYNctl_ver4_etud_obfusc/Systeme non lineaire/Sphere/Subsystem4 ==
  In4 : Inport  Tag=Theta
  Gain : Gain  Gain=-mS*g/(mS+JS/rS^2)
  Integrator : Integrator
  Integrator1 : Integrator
  Out4 : Outport
  Out1 : Outport  Port=2
  Out2 : Outport  Port=3
  wires:
  Gain/1 -> Out2/1, Integrator/1
  In4/1 -> Gain/1
  Integrator1/1 -> Out4/1
  Integrator/1 -> Out1/1, Integrator1/1
